simulink subsystem "PID_and_LQR"  (R2024a)
settings: Solver=VariableStepAuto  StartTime=0.0  StopTime=10.0  RelTol=1e-3
undefined symbols (not defined in the file): z0
settings Model: Creator=Bocchio  LastModifiedBy=Bocchio

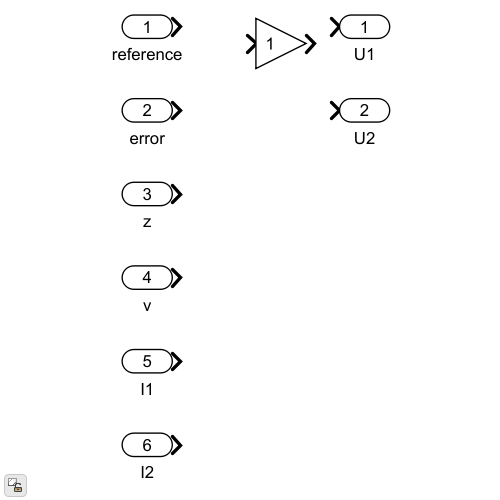
[thumbnail: Simulink's stored preview of the top-level diagram]
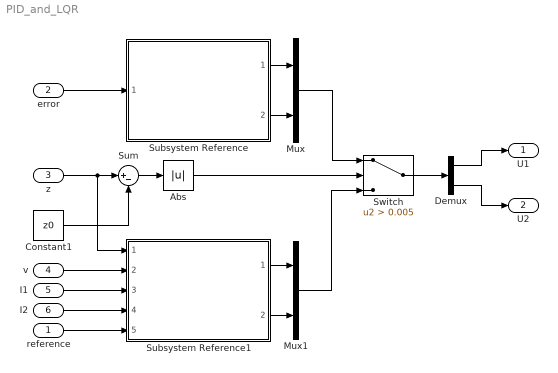
== system PID_and_LQR ==
  reference : Inport
  error : Inport  Port=2
  z : Inport  Port=3
  v : Inport  Port=4
  I1 : Inport  Port=5
  I2 : Inport  Port=6
  Abs : Abs  SaturateOnIntegerOverflow=off
  Constant1 : Constant  Value=z0
  Demux : Demux  Outputs=2
  Mux : Mux  Inputs=2
  Mux1 : Mux  Inputs=2
  Subsystem Reference : Subsystem  ReferencedSubsystem=PID_anti_windup
  Subsystem Reference1 : Subsystem  ReferencedSubsystem=LQR
  Sum : Sum  Inputs=|+-
  Switch : Switch  Criteria=u2 > Threshold  Threshold=0.005  SaturateOnIntegerOverflow=off  InputSameDT=off
  U1 : Outport
  U2 : Outport  Port=2
  wires:
  Demux/2 -> U2/1
  Switch/1 -> Demux/1
  Abs/1 -> Switch/2
  z/1 -> Sum/1, Subsystem Reference1/1
  Constant1/1 -> Sum/2
  Sum/1 -> Abs/1
  Subsystem Reference/1 -> Mux/1
  Subsystem Reference/2 -> Mux/2
  Mux/1 -> Switch/1
  error/1 -> Subsystem Reference/1
  Demux/1 -> U1/1
  Mux1/1 -> Switch/3
  Subsystem Reference1/1 -> Mux1/1
  Subsystem Reference1/2 -> Mux1/2
  reference/1 -> Subsystem Reference1/5
  I2/1 -> Subsystem Reference1/4
  I1/1 -> Subsystem Reference1/3
  v/1 -> Subsystem Reference1/2
